simulink model "Exercise1"  (R2024b)
settings: Solver=ode3  StartTime=0.0  StopTime=10.0  FixedStep=0.01  RelTol=1e-3
settings Model: Creator=balaj  LastModifiedBy=balaj

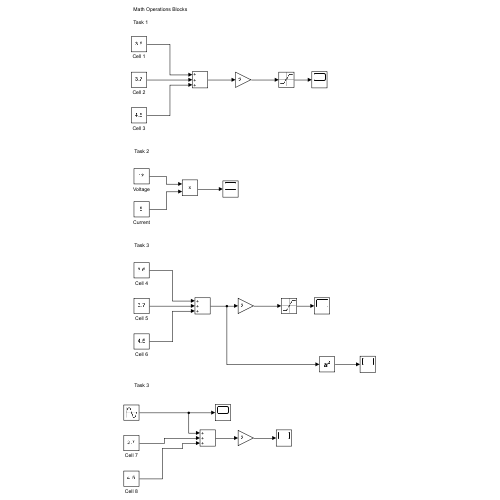
[thumbnail: Simulink's stored preview of the top-level diagram]
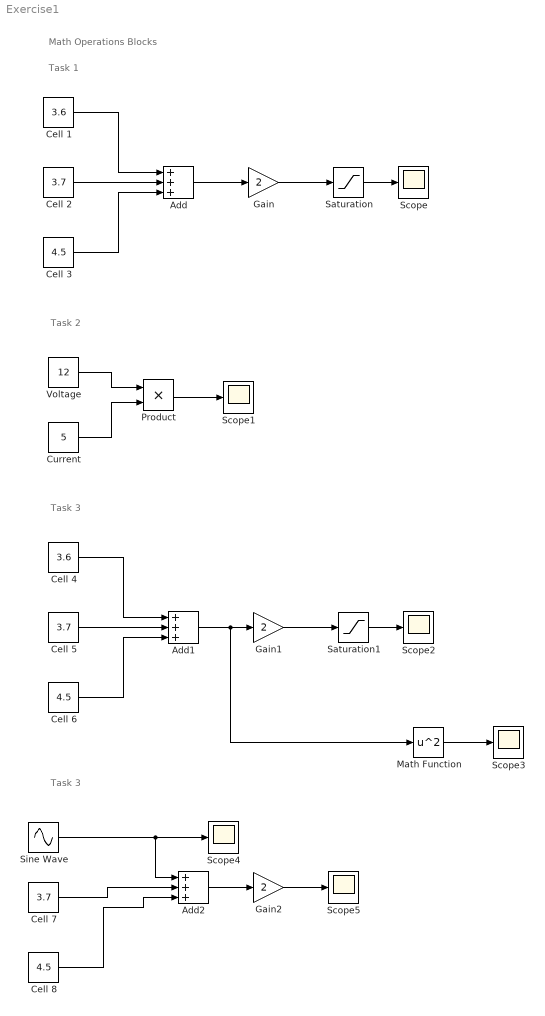
== system Exercise1 ==
  note: Math Operations Blocks
  note: Task 1
  note: Task 2
  note: Task 3
  note: Task 3
  Add : Sum  Inputs=+++
  Add1 : Sum  Inputs=+++
  Add2 : Sum  Inputs=+++
  Cell 1 : Constant  Value=3.6  SampleTime=1
  Cell 2 : Constant  Value=3.7  SampleTime=1
  Cell 3 : Constant  Value=4.5  SampleTime=1
  Cell 4 : Constant  Value=3.6  SampleTime=1
  Cell 5 : Constant  Value=3.7  SampleTime=1
  Cell 6 : Constant  Value=4.5  SampleTime=1
  Cell 7 : Constant  Value=3.7  SampleTime=1
  Cell 8 : Constant  Value=4.5  SampleTime=1
  Current : Constant  Value=5  SampleTime=1
  Gain : Gain  Gain=2
  Gain1 : Gain  Gain=2
  Gain2 : Gain  Gain=2
  Math Function : Math  Operator=square
  Product : Product
  Saturation : Saturate  UpperLimit=12  LowerLimit=0
  Saturation1 : Saturate  UpperLimit=12  LowerLimit=0
  Scope{,1..5} (6 alike) : Scope
  Sine Wave : Sin  Frequency=6.28  SampleTime=0
  Voltage : Constant  Value=12  SampleTime=1
  wires:
  Cell 1/1 -> Add/1
  Cell 2/1 -> Add/2
  Cell 3/1 -> Add/3
  Add/1 -> Gain/1
  Gain/1 -> Saturation/1
  Saturation/1 -> Scope/1
  Voltage/1 -> Product/1
  Current/1 -> Product/2
  Product/1 -> Scope1/1
  Saturation1/1 -> Scope2/1
  Gain1/1 -> Saturation1/1
  Add1/1 -> Math Function/1, Gain1/1
  Cell 6/1 -> Add1/3
  Cell 5/1 -> Add1/2
  Cell 4/1 -> Add1/1
  Math Function/1 -> Scope3/1
  Sine Wave/1 -> Add2/1, Scope4/1
  Cell 7/1 -> Add2/2
  Cell 8/1 -> Add2/3
  Add2/1 -> Gain2/1
  Gain2/1 -> Scope5/1
